simulink model "OldDragModel"  (R2015b)
settings: Solver=VariableStepAuto  StartTime=0.0  StopTime=10.0  RelTol=1e-3
libraries: QuaternionLibrary x1
settings Model: Creator=jban039  LastModifiedBy=jban039

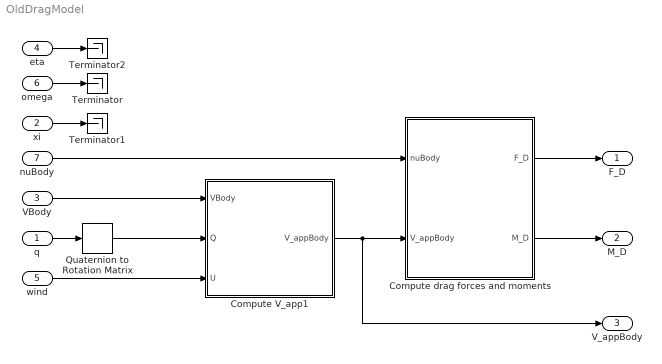
== system OldDragModel ==
  q : Inport  PortDimensions=4
  xi : Inport  Port=2  PortDimensions=3
  VBody : Inport  Port=3  PortDimensions=3
  eta : Inport  Port=4  PortDimensions=3
  wind : Inport  Port=5  PortDimensions=3
  omega : Inport  Port=6  PortDimensions=Uav.N_ROTORS
  nuBody : Inport  Port=7  PortDimensions=3
  Compute V_app1 : MATLAB Function  TreatAsAtomicUnit=on
  Compute drag forces and moments : MATLAB Function  TreatAsAtomicUnit=on
  Quaternion to Rotation Matrix : QuaternionLibrary/Quaternion to Rotation Matrix
  Terminator : Terminator
  Terminator1 : Terminator
  Terminator2 : Terminator
  F_D : Outport
  M_D : Outport  Port=2
  V_appBody : Outport  Port=3
  wires:
  Compute drag forces and moments/1(F_D) -> F_D/1
  Compute drag forces and moments/2(M_D) -> M_D/1
  Compute V_app1/1(V_appBody) -> V_appBody/1, Compute drag forces and moments/2(V_appBody)
  omega/1 -> Terminator/1
  xi/1 -> Terminator1/1
  nuBody/1 -> Compute drag forces and moments/1(nuBody)
  VBody/1 -> Compute V_app1/1(VBody)
  q/1 -> Quaternion to Rotation Matrix/1
  Quaternion to Rotation Matrix/1 -> Compute V_app1/2(Q)
  wind/1 -> Compute V_app1/3(U)
  eta/1 -> Terminator2/1

== matlab function OldDragModel/Compute drag forces and moments ==
  data: nuBody input; V_appBody input; F_D output; M_D output; Uav parameter
function [F_D, M_D] = computeDrag(nuBody, V_appBody, Uav)
%#codegen

% Calculate drag force
F_D = 0.5 * Uav.RHO_AIR * Uav.C_D * (norm(V_appBody) .* V_appBody);

% Drag moment, applied to independent axes
M_D = 0.5 * Uav.RHO_AIR * Uav.C_DM * (norm(nuBody) .* nuBody);

== matlab function OldDragModel/Compute V_app1 ==
  data: VBody input; Q input; V_appBody output; U input size=3
function V_appBody = computeV_appBody(VBody, Q, U)
%#codegen

% Rotation matrix from Wind frame to Inertial frame 
R_U = [1, 0,  0;
       0, 1,  0;
       0, 0, -1];

V_appBody = VBody + Q'*R_U*U;
